simulink model "block_propagator"  (R2019b)
settings: Solver=FixedStepAuto  StartTime=0.0  StopTime=10.0  RelTol=1e-3
undefined symbols (not defined in the file or in its folder): __PRM__SERIALIZED__DATA__, SubsystemReferenceBlock, w0
libraries: blocklib x1
settings Model: Creator=Imanol  LastModifiedBy=imanol
settings SFSimCC: CustomCodeUndefinedFunction=UseInterfaceOnly

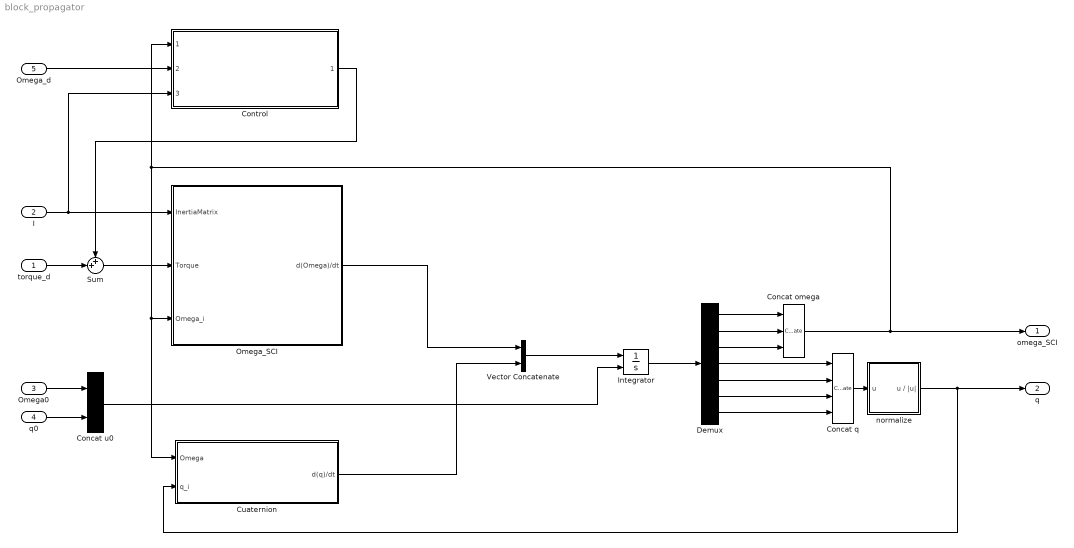
== system block_propagator ==
  torque_d : Inport  Unit=N*m  PortDimensions=[3,1]
  I : Inport  Port=2  Unit=kg*m*m*m*m  PortDimensions=[3,3]
  Omega0 : Inport  Port=3  Unit=rad/sec  PortDimensions=[3,1]
  q0 : Inport  Port=4  PortDimensions=[4,1]
  Omega_d : Inport  Port=5  Unit=rad/sec  PortDimensions=[3,1]
  Concat omega : Concatenate  NumInputs=3
  Concat q : Concatenate  NumInputs=4
  Concat u0 : Concatenate
  Control : Subsystem  BlockKeywords=__PRM__SERIALIZED__DATA__:SubsystemReferenceBlock  ReferencedSubsystem=block_control
  Cuaternion : Subsystem
  Demux : Demux  Outputs=7
  Integrator : Integrator  InitialConditionSource=external  InitialCondition=w0  ContinuousStateAttributes='attitude'
  Omega_SCI : Subsystem
  Sum : Sum  Inputs=++|
  Vector Concatenate : Concatenate
  normalize : Subsystem
  omega_SCI : Outport  VectorParamsAs1DForOutWhenUnconnected=off
  q : Outport  Port=2  VectorParamsAs1DForOutWhenUnconnected=off
  wires:
  Cuaternion/1(d(q)/dt) -> Vector Concatenate/2
  Sum/1 -> Omega_SCI/2(Torque)
  I/1 -> Control/3, Omega_SCI/1(InertiaMatrix)
  Omega_SCI/1(d(Omega)/dt) -> Vector Concatenate/1
  Omega0/1 -> Concat u0/1
  q0/1 -> Concat u0/2
  Vector Concatenate/1 -> Integrator/1
  Concat u0/1 -> Integrator/2
  Integrator/1 -> Demux/1
  Demux/1 -> Concat omega/1
  Demux/2 -> Concat omega/2
  Demux/3 -> Concat omega/3
  Demux/4 -> Concat q/1
  Demux/5 -> Concat q/2
  Demux/6 -> Concat q/3
  Demux/7 -> Concat q/4
  Concat omega/1 -> Control/1, Omega_SCI/3(Omega_i), Cuaternion/1(Omega), omega_SCI/1
  Concat q/1 -> normalize/1(u)
  normalize/1(u / |u|) -> Cuaternion/2(q_i), q/1
  Control/1 -> Sum/1
  torque_d/1 -> Sum/2
  Omega_d/1 -> Control/2

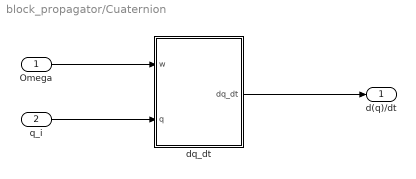
== system block_propagator/Cuaternion ==
  Omega : Inport
  q_i : Inport  Port=2
  dq_dt : MATLAB Function  TreatAsAtomicUnit=on
  d(q)/dt : Outport  VectorParamsAs1DForOutWhenUnconnected=off
  wires:
  Omega/1 -> dq_dt/1(w)
  q_i/1 -> dq_dt/2(q)
  dq_dt/1(dq_dt) -> d(q)/dt/1

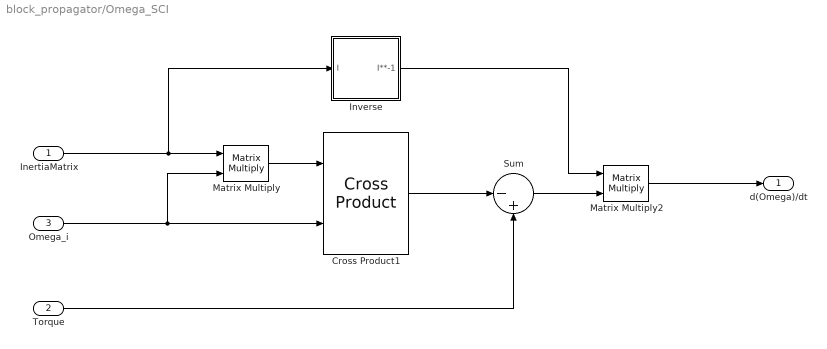
== system block_propagator/Omega_SCI ==
  InertiaMatrix : Inport
  Torque : Inport  Port=2
  Omega_i : Inport  Port=3
  Cross Product1 : blocklib/Cross Product  SystemSampleTime=-1  Latency=0  AutoFrameSizeCalculation=off
      settings: SourceProductName=Custom Library
  Inverse : Subsystem
  Matrix Multiply : Product  Multiplication=Matrix(*)
  Matrix Multiply2 : Product  Multiplication=Matrix(*)
  Sum : Sum  Inputs=|-+
  d(Omega)/dt : Outport  VectorParamsAs1DForOutWhenUnconnected=off
  wires:
  Cross Product1/1 -> Sum/1
  Omega_i/1 -> Cross Product1/2, Matrix Multiply/2
  Torque/1 -> Sum/2
  Sum/1 -> Matrix Multiply2/2
  InertiaMatrix/1 -> Inverse/1(I), Matrix Multiply/1
  Matrix Multiply/1 -> Cross Product1/1
  Matrix Multiply2/1 -> d(Omega)/dt/1
  Inverse/1(I**-1) -> Matrix Multiply2/1

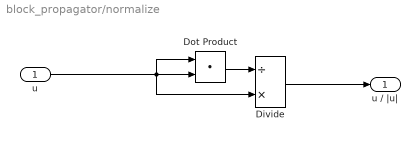
== system block_propagator/normalize ==
  u : Inport
  Divide : Product  Inputs=/*
  Dot Product : DotProduct  InputSameDT=on  OutDataTypeStr=Inherit: Inherit via internal rule
  u / |u| : Outport
  wires:
  Dot Product/1 -> Divide/1
  u/1 -> Dot Product/1, Divide/2, Dot Product/2
  Divide/1 -> u / |u|/1

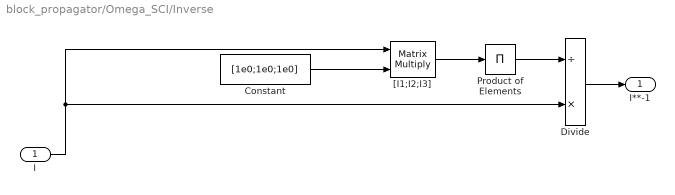
== system block_propagator/Omega_SCI/Inverse ==
  I : Inport
  Constant : Constant  Value=[1e0;1e0;1e0]
  Divide : Product  Inputs=/*
  Product of Elements : Product  Inputs=*
  "[I1;I2;I3]" : Product  Multiplication=Matrix(*)
  I**-1 : Outport
  wires:
  "[I1;I2;I3]"/1 -> Product of Elements/1
  Divide/1 -> I**-1/1
  Product of Elements/1 -> Divide/1
  I/1 -> Divide/2, "[I1;I2;I3]"/1
  Constant/1 -> "[I1;I2;I3]"/2

== matlab function block_propagator/Cuaternion/dq_dt ==
  data: w input; dq_dt output; q input
function dq_dt = fcn(w, q)
mat = zeros(4, 4);
mat(1:3, 1:3) = - [0. -w(3) w(2) ; w(3) 0. -w(1) ; -w(2) w(1) 0. ];
mat(1:3, 4) = w;
mat(4, 1:3) = -w';
mat(4, 4) = 0.;
dq_dt = 5e-1 * mat * q;
